simulink model "sim_thruster_wsim_hrn"  (R2014b)
settings: Solver=FixedStepDiscrete  StartTime=t0  StopTime=tFinal  FixedStep=sim_dt  RelTol=1e-3
libraries: csc_valvesim_sim_lib x1, csu_cfe_cfe_time_lib x1, csu_tdl_thruster_dynamics_lander_lib x1
settings Model: Creator=escrane  LastModifiedBy=mstewart
settings DebuggingCC: UnderspecifiedInitializationDetection=Classic  MergeDetectMultiDrivingBlocksExec=none

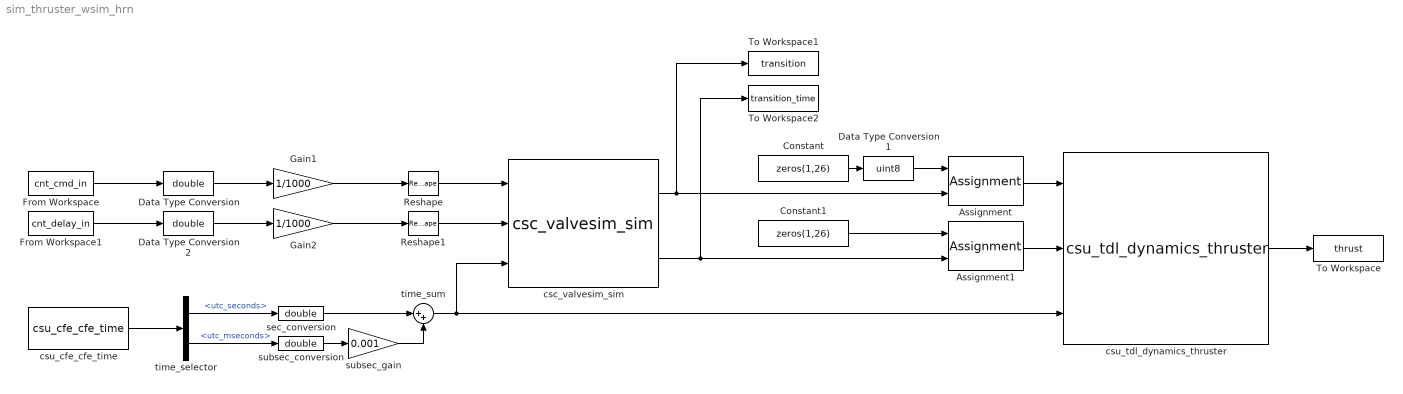
== system sim_thruster_wsim_hrn ==
  Assignment : Assignment  Indices=test_thruster_id
  Assignment1 : Assignment  Indices=test_thruster_id
  Constant : Constant  Value=zeros(1,26)
  Constant1 : Constant  Value=zeros(1,26)
  Data Type Conversion : DataTypeConversion  OutDataTypeStr=double
  Data Type Conversion1 : DataTypeConversion  OutDataTypeStr=uint8
  Data Type Conversion2 : DataTypeConversion  OutDataTypeStr=double
  From Workspace : FromWorkspace  VariableName=cnt_cmd_in  SampleTime=0
  From Workspace1 : FromWorkspace  VariableName=cnt_delay_in  SampleTime=0
  Gain1 : Gain  Gain=1/1000  OutDataTypeStr=double
  Gain2 : Gain  Gain=1/1000  OutDataTypeStr=double
  Reshape : Reshape
  Reshape1 : Reshape
  To Workspace : ToWorkspace  VariableName=thrust  SaveFormat=Timeseries  SampleTime=-1
  To Workspace1 : ToWorkspace  VariableName=transition  SaveFormat=Timeseries  SampleTime=-1
  To Workspace2 : ToWorkspace  VariableName=transition_time  SaveFormat=Timeseries  SampleTime=-1
  csc_valvesim_sim : csc_valvesim_sim_lib/csc_valvesim_sim  thruster_idx=test_thruster_id
  csu_cfe_cfe_time : csu_cfe_cfe_time_lib/csu_cfe_cfe_time  sch_dt=sim_time_step_size
  csu_tdl_dynamics_thruster : csu_tdl_thruster_dynamics_lander_lib/csu_tdl_dynamics_thruster  thruster_idx=test_thruster_id  time_since_rise_lookup=tdl_thruster1_rising_lookup_time  thrust_rising_output_lookup=tdl_thruster1_rising_lookup_thrust  time_since_fall_lookup=tdl_thruster1_falling_lookup_time  thrust_falling_output_lookup=tdl_thruster1_falling_lookup_thrust  thrust_noise_mean=tdl_thruster1_thrust_noise_mean  thrust_noise_std=tdl_thruster1_thrust_noise_std  thrust_noise_seed=tdl_thruster1_thrust_noise_seed  thrust_noise_on=0
  sec_conversion : DataTypeConversion  OutDataTypeStr=double  SaturateOnIntegerOverflow=on  RndMeth=Zero
  subsec_conversion : DataTypeConversion  OutDataTypeStr=double  SaturateOnIntegerOverflow=on  RndMeth=Zero
  subsec_gain : Gain  Gain=0.001  SaturateOnIntegerOverflow=on  OutDataTypeStr=Inherit: Same as input  ParamDataTypeStr=Inherit: Same as input
  time_selector : BusSelector  OutputSignals=utc_seconds,utc_mseconds
  time_sum : Sum  Inputs=|++  SaturateOnIntegerOverflow=on  InputSameDT=on  OutDataTypeStr=Inherit: Same as first input
  wires:
  csu_tdl_dynamics_thruster/1 -> To Workspace/1
  Data Type Conversion/1 -> Gain1/1
  From Workspace/1 -> Data Type Conversion/1
  time_sum/1 -> csc_valvesim_sim/3, csu_tdl_dynamics_thruster/3
  sec_conversion/1 -> time_sum/1
  subsec_gain/1 -> time_sum/2
  subsec_conversion/1 -> subsec_gain/1
  time_selector/2 -> subsec_conversion/1  "<utc_mseconds>"
  time_selector/1 -> sec_conversion/1  "<utc_seconds>"
  csu_cfe_cfe_time/1 -> time_selector/1
  Gain1/1 -> Reshape/1
  Reshape/1 -> csc_valvesim_sim/1
  csc_valvesim_sim/1 -> To Workspace1/1, Assignment/2
  Assignment/1 -> csu_tdl_dynamics_thruster/1
  Assignment1/1 -> csu_tdl_dynamics_thruster/2
  csc_valvesim_sim/2 -> To Workspace2/1, Assignment1/2
  Constant/1 -> Data Type Conversion1/1
  Constant1/1 -> Assignment1/1
  Data Type Conversion1/1 -> Assignment/1
  Data Type Conversion2/1 -> Gain2/1
  From Workspace1/1 -> Data Type Conversion2/1
  Gain2/1 -> Reshape1/1
  Reshape1/1 -> csc_valvesim_sim/2
